simulink model "propeller"  (R2019b)
settings: Solver=VariableStepAuto  StartTime=0.0  StopTime=180  MaxStep=1e-2  RelTol=1e-3
undefined symbols (not defined in the file or in its folder): X, Y, Z
libraries: sm_lib x26, cstblocks x23, nesl_utility x20, simulink x2
(part 1 of 3)
settings Model: PauseTimes=1.42  EnablePacing=on  Creator=lenovo  LastModifiedBy=lenovo

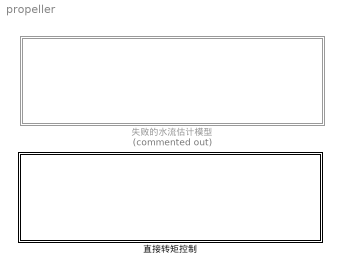
== system propeller ==
  失败的水流估计模型 : Subsystem  Commented=on
  直接转矩控制 : Subsystem

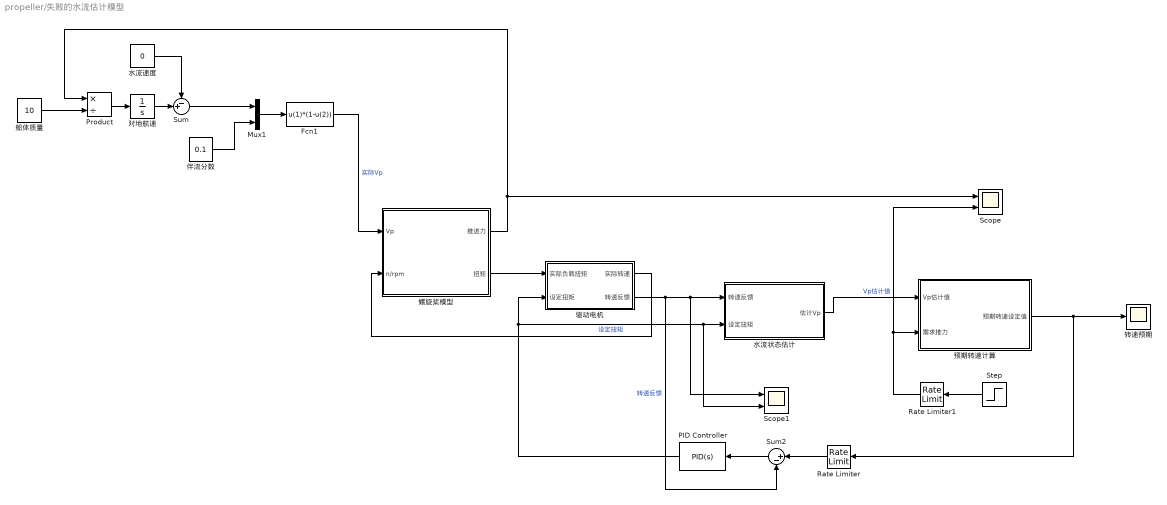
== system propeller/失败的水流估计模型 ==
  Fcn1 : Fcn  Expr=u(1)*(1-u(2))
  Mux1 : Mux  Inputs=2
  PID Controller : simulink/Continuous/PID Controller  Controller=PID  Form=Parallel  TimeDomain=Continuous-time  SampleTime=-1  IntegratorMethod=Forward Euler  FilterMethod=Forward Euler  ControllerParametersSource=internal  P=0.05  I=0.01  D=0  UseFilter=on  N=100  TunerSelectOption=Transfer Function Based (PID Tuner App)  InitialConditionSource=internal  InitialConditionForIntegrator=0  InitialConditionForFilter=0  DifferentiatorICPrevScaledInput=0  ExternalReset=none  TrackingMode=off  Kt=1  LimitOutput=on  UpperSaturationLimit=250  LowerSaturationLimit=-250  LinearizeAsGain=on  AntiWindupMode=none  Kb=1  POutMin=[]  POutMax=[]  IOutMin=[]  IOutMax=[]  DOutMin=[]  DOutMax=[]  NOutMin=[]  NOutMax=[]  SumOutMin=[]  SumOutMax=[]  SaturationOutMin=[]  SaturationOutMax=[]  PParamMin=[]  PParamMax=[]  IParamMin=[]  IParamMax=[]  DParamMin=[]  DParamMax=[]  NParamMin=[]  NParamMax=[]  KbParamMin=[]  KbParamMax=[]  KtParamMin=[]  KtParamMax=[]  KbOutMin=[]  KbOutMax=[]  KtOutMin=[]  KtOutMax=[]  IntegratorOutMin=[]  IntegratorOutMax=[]  FilterOutMin=[]  FilterOutMax=[]  SumI1OutMin=[]  SumI1OutMax=[]  SumI2OutMin=[]  SumI2OutMax=[]  SumI3OutMin=[]  SumI3OutMax=[]  SumI4OutMin=[]  SumI4OutMax=[]  SumDOutMin=[]  SumDOutMax=[]  DifferentiatorOutMin=[]  DifferentiatorOutMax=[]  FilterDiffOutCoefMin=[]  FilterDiffOutCoefMax=[]  ReciprocalOutMin=[]  ReciprocalOutMax=[]  SumDenOutMin=[]  SumDenOutMax=[]  SumNumOutMin=[]  SumNumOutMax=[]  DivideOutMin=[]  DivideOutMax=[]  IntegratorContinuousStateAttributes=''  IntegratorStateMustResolveToSignalObject=off  IntegratorRTWStateStorageClass=Auto  FilterContinuousStateAttributes=''  FilterStateMustResolveToSignalObject=off  FilterRTWStateStorageClass=Auto  ParallelPVariant=InternalParameters  IdealPVariant=Disabled  IVariant=InternalParameters  DVariant=InternalParameters  IntegratorVariant=Continuous  SatVariant=Enabled  AWVariant=Passthrough  PCopyVariant=Disabled  TRVariant=Disabled  FdbkBlocksVariant=Forward  IdealPFdbkVariant=Disabled  SatFdbkVariant=Disabled  DerivativeFilterVariant=ContFilter  NVariant=InternalParameters  NCopyVariant=Disabled  FilterICVariant=InternalICsFilter  IntegratorICVariant=InternalICs  ExternalResetVariant=Disabled  TRSumVariant=Passthrough  SumFdbkVariant=Disabled  SumVariant=Sum_PID
  Product : Product  Inputs=*/
  Rate Limiter : RateLimiter  RisingSlewLimit=200  FallingSlewLimit=-200  SampleTimeMode=inherited
  Rate Limiter1 : RateLimiter  RisingSlewLimit=3  FallingSlewLimit=-3  SampleTimeMode=inherited
  Scope : Scope  NumInputPorts=2
  Scope1 : Scope  NumInputPorts=2
  Step : Step  Time=5  Before=1  After=3  SampleTime=0
  Sum : Sum  Inputs=-+|
  Sum2 : Sum  Inputs=|+-
  伴流分数 : Constant  Value=0.1
  对地航速 : Integrator
  水流状态估计 : Subsystem
  水流速度 : Constant  Value=0
  船体质量 : Constant  Value=10
  螺旋桨模型 : Subsystem  mask{rou_Set=1.023, D_Set=1}
      mask prompts: rou_Set "海水密度 g/cm3 (rou_Set)"; D_Set "螺旋桨直径 D_Set"
  转速预期 : Scope
  预期转速计算 : Subsystem
  驱动电机 : Subsystem  mask{Trq_Max=250, Spe_Max=20000, J_Set=0.1}
      mask prompts: Trq_Max "电机最大扭矩"; Spe_Max "电机最高转速"; J_Set "系统转动惯量"
  wires:
  驱动电机/2(转速反馈) -> Sum2/2, Scope1/1, 水流状态估计/1(转速反馈)  "转速反馈"
  PID Controller/1 -> 驱动电机/2(设定扭矩), Scope1/2, 水流状态估计/2(设定扭矩)  "设定扭矩"
  螺旋桨模型/2(扭矩) -> 驱动电机/1(实际负载扭矩)
  Product/1 -> 对地航速/1
  Rate Limiter1/1 -> Scope/2, 预期转速计算/2(需求推力)
  水流状态估计/1(估计Vp) -> 预期转速计算/1(Vp估计值)  "Vp估计值"
  驱动电机/1(实际转速) -> 螺旋桨模型/2(n/rpm)
  Sum/1 -> Mux1/1
  Sum2/1 -> PID Controller/1
  Fcn1/1 -> 螺旋桨模型/1(Vp)  "实际Vp"
  Step/1 -> Rate Limiter1/1
  对地航速/1 -> Sum/2
  Rate Limiter/1 -> Sum2/1
  预期转速计算/1(预期转速设定值) -> Rate Limiter/1, 转速预期/1
  螺旋桨模型/1(推进力) -> Product/1, Scope/1
  Mux1/1 -> Fcn1/1
  伴流分数/1 -> Mux1/2
  船体质量/1 -> Product/2
  水流速度/1 -> Sum/1

== system propeller/直接转矩控制 ==
  Constant2 : Constant  Value=60
  Constant3 : Constant  Value=2.5
  GPS船速 : Subsystem
  Rate Limiter1 : RateLimiter  RisingSlewLimit=2  FallingSlewLimit=-2  SampleTimeMode=inherited
  Slider : SliderBlock  ScaleMin=-60  ScaleMax=60
  保证初始设定值为0 : TransportDelay  DelayTime=0.01
  船体、水体物理模型 : Subsystem
  船速、朝向控制器 : Subsystem
  wires:
  GPS船速/1(纵向速度) -> 船速、朝向控制器/5(前进速度反馈)
  GPS船速/2(横向速度) -> 船速、朝向控制器/6(侧移速度反馈)
  船体、水体物理模型/3(Angle) -> 船速、朝向控制器/7(角度反馈), GPS船速/3(Alpha)
  船速、朝向控制器/1(左推进方向) -> 船体、水体物理模型/1(左推进方向设定)
  船速、朝向控制器/2(右推进方向) -> 船体、水体物理模型/2(右推进方向设定)
  船速、朝向控制器/3(左电机扭矩) -> 船体、水体物理模型/3(左设定扭矩)
  船速、朝向控制器/4(右电机扭矩) -> 船体、水体物理模型/4(右设定扭矩)
  船体、水体物理模型/4(左转速反馈) -> 船速、朝向控制器/1(左电机转速反馈)
  船体、水体物理模型/5(实际推进方向) -> 船速、朝向控制器/2(推进方向反馈)
  船体、水体物理模型/6(右转速反馈) -> 船速、朝向控制器/3(右电机转速反馈)
  船体、水体物理模型/7(wz) -> 船速、朝向控制器/4(角速度反馈)
  船体、水体物理模型/8(Vx) -> GPS船速/1(Vx)
  船体、水体物理模型/9(Vy) -> GPS船速/2(Vy)
  Rate Limiter1/1 -> 船速、朝向控制器/8(船头方向设定)
  Constant2/1 -> 保证初始设定值为0/1
  保证初始设定值为0/1 -> Rate Limiter1/1
  Constant3/1 -> 船速、朝向控制器/9(前进速度设定)

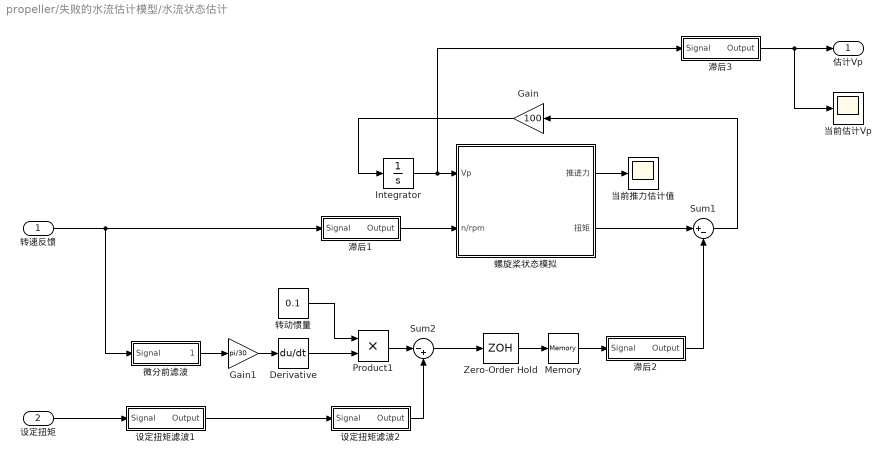
== system propeller/失败的水流估计模型/水流状态估计 ==
  转速反馈 : Inport
  设定扭矩 : Inport  Port=2
  Derivative : Derivative  CoefficientInTFapproximation=1/25
  Gain : Gain  Gain=100
  Gain1 : Gain  Gain=pi/30
  Integrator : Integrator  LimitOutput=on  UpperSaturationLimit=20  LowerSaturationLimit=-20
  Memory : Memory
  Product1 : Product
  Sum1 : Sum  Inputs=|+-
  Sum2 : Sum  Inputs=|-+
  Zero-Order Hold : ZeroOrderHold  SampleTime=0.01
  当前估计Vp : Scope
  当前推力估计值 : Scope
  微分前滤波 : Subsystem  mask{Frq=10, Order=1}
      mask prompts: Frq "Frq_Set"; Order "Order_Set"
  滞后1 : Subsystem  mask{Frq=5, Order=1}
      mask prompts: Frq "Frq_Set"; Order "Order_Set"
  滞后2 : Subsystem  mask{Frq=5, Order=1}
      mask prompts: Frq "Frq_Set"; Order "Order_Set"
  滞后3 : Subsystem  mask{Frq=2, Order=10}
      mask prompts: Frq "Frq_Set"; Order "Order_Set"
  螺旋桨状态模拟 : Subsystem  mask{rou_Set=1.023, D_Set=1}
      mask prompts: rou_Set "海水密度 g/cm3 (rou_Set)"; D_Set "螺旋桨直径 D_Set"
  设定扭矩滤波1 : Subsystem  mask{Frq=25, Order=1}
      mask prompts: Frq "Frq_Set"; Order "Order_Set"
  设定扭矩滤波2 : Subsystem  mask{Frq=10, Order=1}
      mask prompts: Frq "Frq_Set"; Order "Order_Set"
  转动惯量 : Constant  Value=0.1
  估计Vp : Outport
  wires:
  微分前滤波/1(Output) -> Gain1/1
  Gain1/1 -> Derivative/1
  Product1/1 -> Sum2/1
  螺旋桨状态模拟/2(扭矩) -> Sum1/1
  转速反馈/1 -> 微分前滤波/1(Signal), 滞后1/1(Signal)
  滞后2/1(Output) -> Sum1/2
  转动惯量/1 -> Product1/1
  Derivative/1 -> Product1/2
  滞后1/1(Output) -> 螺旋桨状态模拟/2(n/rpm)
  螺旋桨状态模拟/1(推进力) -> 当前推力估计值/1
  设定扭矩滤波1/1(Output) -> 设定扭矩滤波2/1(Signal)
  Gain/1 -> Integrator/1
  设定扭矩滤波2/1(Output) -> Sum2/2
  滞后3/1(Output) -> 当前估计Vp/1, 估计Vp/1
  Sum2/1 -> Zero-Order Hold/1
  设定扭矩/1 -> 设定扭矩滤波1/1(Signal)
  Sum1/1 -> Gain/1
  Integrator/1 -> 滞后3/1(Signal), 螺旋桨状态模拟/1(Vp)
  Zero-Order Hold/1 -> Memory/1
  Memory/1 -> 滞后2/1(Signal)

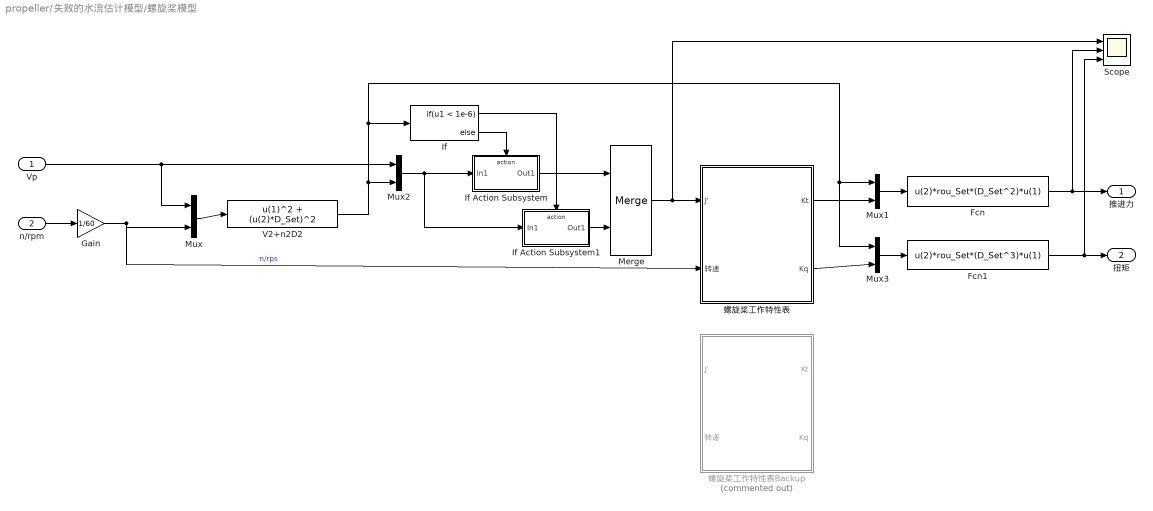
== system propeller/失败的水流估计模型/螺旋桨模型 ==
  Vp : Inport
  n/rpm : Inport  Port=2
  Fcn : Fcn  Expr=u(2)*rou_Set*(D_Set^2)*u(1)
  Fcn1 : Fcn  Expr=u(2)*rou_Set*(D_Set^3)*u(1)
  Gain : Gain  Gain=1/60
  If : If  IfExpression=u1 < 1e-6
  If Action Subsystem : Subsystem  TreatAsAtomicUnit=on
  If Action Subsystem1 : Subsystem  TreatAsAtomicUnit=on
  Merge : Merge
  Mux{,1..3} (4 alike) : Mux  Inputs=2
  Scope : Scope  NumInputPorts=3
  V2+n2D2 : Fcn  Expr=u(1)^2 + (u(2)*D_Set)^2
  螺旋桨工作特性表 : Subsystem
  螺旋桨工作特性表Backup : Subsystem  Commented=on
  推进力 : Outport
  扭矩 : Outport  Port=2
  wires:
  Mux2/1 -> If Action Subsystem1/1(In1), If Action Subsystem/1(In1)
  n/rpm/1 -> Gain/1
  Vp/1 -> Mux2/1, Mux/1
  If/2 -> If Action Subsystem/Action
  If Action Subsystem/1(Out1) -> Merge/1
  Gain/1 -> 螺旋桨工作特性表/2(转速), Mux/2  "n/rps"
  If/1 -> If Action Subsystem1/Action
  If Action Subsystem1/1(Out1) -> Merge/2
  Mux/1 -> V2+n2D2/1
  Merge/1 -> Scope/1, 螺旋桨工作特性表/1(J')
  螺旋桨工作特性表/1(Kt) -> Mux1/2
  螺旋桨工作特性表/2(Kq) -> Mux3/2
  Mux1/1 -> Fcn/1
  V2+n2D2/1 -> If/1, Mux3/1, Mux1/1, Mux2/2
  Mux3/1 -> Fcn1/1
  Fcn1/1 -> Scope/3, 扭矩/1
  Fcn/1 -> Scope/2, 推进力/1

== system propeller/失败的水流估计模型/预期转速计算 ==
  Vp估计值 : Inport
  需求推力 : Inport  Port=2
  Gain : Gain  Gain=1000
  Integrator : Integrator
  Sum1 : Sum  Inputs=+-|
  当前扭矩估计值 : Scope
  滞后2 : Subsystem  mask{Frq=0.2, Order=5}
      mask prompts: Frq "Frq_Set"; Order "Order_Set"
  螺旋桨状态模拟 : Subsystem  mask{rou_Set=1.023, D_Set=1}
      mask prompts: rou_Set "海水密度 g/cm3 (rou_Set)"; D_Set "螺旋桨直径 D_Set"
  预期转速设定值 : Outport
  wires:
  螺旋桨状态模拟/1(推进力) -> Sum1/2
  Gain/1 -> Integrator/1
  Integrator/1 -> 滞后2/1(Signal), 螺旋桨状态模拟/2(n/rpm)
  Sum1/1 -> Gain/1
  螺旋桨状态模拟/2(扭矩) -> 当前扭矩估计值/1
  需求推力/1 -> Sum1/1
  Vp估计值/1 -> 螺旋桨状态模拟/1(Vp)
  滞后2/1(Output) -> 预期转速设定值/1

== system propeller/失败的水流估计模型/驱动电机 ==
  实际负载扭矩 : Inport
  设定扭矩 : Inport  Port=2
  Gain : Gain  Gain=30/pi
  Integrator : Integrator  LimitOutput=on  UpperSaturationLimit=5000  LowerSaturationLimit=-5000
  Product1 : Product  Inputs=/*
  Saturation : Saturate  UpperLimit=Trq_Max  LowerLimit=-Trq_Max
  Sum1 : Sum  Inputs=|+-
  传感器量化 : Quantizer  QuantizationInterval=Spe_Max/10000
  反馈量滤波 : Subsystem  mask{Frq=25, Order=3}
      mask prompts: Frq "Frq_Set"; Order "Order_Set"
  滞后 : Subsystem  mask{Frq=500, Order=2}
      mask prompts: Frq "Frq_Set"; Order "Order_Set"
  转动惯量 : Constant  Value=J_Set
  通信量化 : Quantizer  QuantizationInterval=Trq_Max/5000
  通信间隔 : ZeroOrderHold  SampleTime=0.01
  实际转速 : Outport
  转速反馈 : Outport  Port=2
  wires:
  通信量化/1 -> Saturation/1
  Sum1/1 -> Product1/2
  通信间隔/1 -> 反馈量滤波/1(Signal)
  传感器量化/1 -> 通信间隔/1
  转动惯量/1 -> Product1/1
  实际负载扭矩/1 -> Sum1/2
  Saturation/1 -> 滞后/1(Signal)
  Product1/1 -> Integrator/1
  滞后/1(Output) -> Sum1/1
  Integrator/1 -> Gain/1  "n_Radps"
  设定扭矩/1 -> 通信量化/1
  反馈量滤波/1(Output) -> 转速反馈/1
  Gain/1 -> 实际转速/1, 传感器量化/1

== system propeller/直接转矩控制/GPS船速 ==
  Vx : Inport
  Vy : Inport  Port=2
  Alpha : Inport  Port=3
  Fcn1 : Fcn  Expr=u(2)*cos(u(3))-u(1)*sin(u(3))
  Fcn2 : Fcn  Expr=u(2)*sin(u(3))+u(1)*cos(u(3))
  Mux1 : Mux  Inputs=3
  传感器量化 : Quantizer  QuantizationInterval=0.01
  传感器量化1 : Quantizer  QuantizationInterval=0.01
  反馈量滤波 : Subsystem  mask{Frq=1, Order=3}
      mask prompts: Frq "Frq_Set"; Order "Order_Set"
  反馈量滤波1 : Subsystem  mask{Frq=1, Order=3}
      mask prompts: Frq "Frq_Set"; Order "Order_Set"
  通信间隔 : ZeroOrderHold  SampleTime=0.01
  通信间隔1 : ZeroOrderHold  SampleTime=0.01
  纵向速度 : Outport
  横向速度 : Outport  Port=2
  wires:
  Fcn1/1 -> 传感器量化/1
  Alpha/1 -> Mux1/3
  Vx/1 -> Mux1/1
  Vy/1 -> Mux1/2
  Mux1/1 -> Fcn1/1, Fcn2/1
  传感器量化/1 -> 通信间隔/1
  反馈量滤波/1(Output) -> 纵向速度/1
  通信间隔/1 -> 反馈量滤波/1(Signal)
  通信间隔1/1 -> 反馈量滤波1/1(Signal)
  传感器量化1/1 -> 通信间隔1/1
  Fcn2/1 -> 传感器量化1/1
  反馈量滤波1/1(Output) -> 横向速度/1

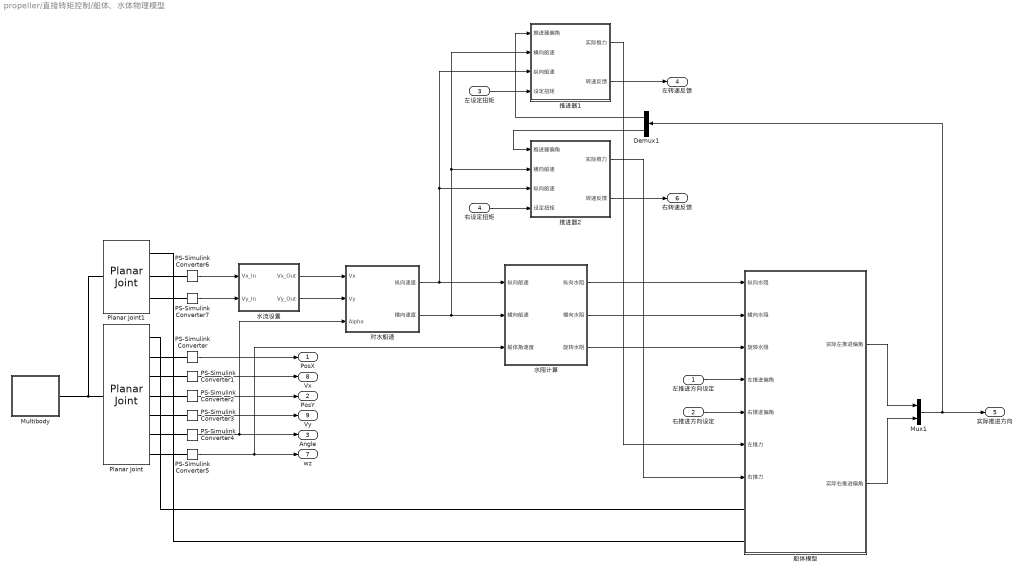
== system propeller/直接转矩控制/船体、水体物理模型 ==
  左推进方向设定 : Inport
  右推进方向设定 : Inport  Port=2
  左设定扭矩 : Inport  Port=3
  右设定扭矩 : Inport  Port=4
  Demux1 : Demux  Outputs=2
  Multibody : Subsystem
  Mux1 : Mux  Inputs=2
  PS-Simulink Converter{,1..7} (8 alike) : nesl_utility/PS-Simulink Converter  PhysicalDomain=network_engine_domain  SubClassName=ps_output  LeftPortType=input  RightPortType=output  PseudoPeriodic=off  Frequencies=[]  Unit=inherit  AffineConversion=off
  Planar Joint : sm_lib/Joints/Planar Joint  JointMode=Normal  SenseConstraintForce=off  SenseConstraintForceX=off  SenseConstraintForceY=off  SenseConstraintForceZ=off  SenseConstraintTorque=off  SenseConstraintTorqueX=off  SenseConstraintTorqueY=off  SenseConstraintTorqueZ=off  SenseTotalForce=off  SenseTotalForceX=off  SenseTotalForceY=off  SenseTotalForceZ=off  SenseTotalTorque=off  SenseTotalTorqueX=off  SenseTotalTorqueY=off  SenseTotalTorqueZ=off  CompositeWrenchDir=FollowerOnBase  CompositeWrenchFrame=BaseFrame  PxEquilibriumPosition=0  PxEquilibriumPositionUnits=m  PxSpringStiffness=0  PxSpringStiffnessUnits=N/m  PxDampingCoefficient=0  PxDampingCoefficientUnits=N/(m/s)  PxTorqueActuationMode=NoTorque  PxMotionActuationMode=ComputedMotion  PxSensePosition=on  PxSenseVelocity=on  PxSenseAcceleration=off  PxSenseTorqueForce=off  PxSenseLowerLimitTorqueForce=off  PxSenseUpperLimitTorqueForce=off  PxLowerLimitSpecify=off  PxLowerLimitBound=-1  PxLowerLimitBoundUnits=m  PxLowerLimitStiffness=1e6  PxLowerLimitStiffnessUnits=N/m  PxLowerLimitDamping=1e3  PxLowerLimitDampingUnits=N/(m/s)  PxLowerLimitTransitionRegionWidth=1e-4  PxLowerLimitTransitionRegionWidthUnits=m  PxUpperLimitSpecify=off  PxUpperLimitBound=1  PxUpperLimitBoundUnits=m  PxUpperLimitStiffness=1e6  PxUpperLimitStiffnessUnits=N/m  PxUpperLimitDamping=1e3  PxUpperLimitDampingUnits=N/(m/s)  PxUpperLimitTransitionRegionWidth=1e-4  PxUpperLimitTransitionRegionWidthUnits=m  PxPositionTargetSpecify=off  PxPositionTargetPriority=High  PxPositionTargetValue=0  PxPositionTargetValueUnits=m  PxVelocityTargetSpecify=off  PxVelocityTargetPriority=High  PxVelocityTargetValue=3  PxVelocityTargetValueUnits=m/s  PyEquilibriumPosition=0  PyEquilibriumPositionUnits=m  PySpringStiffness=0  PySpringStiffnessUnits=N/m  PyDampingCoefficient=0  PyDampingCoefficientUnits=N/(m/s)  PyTorqueActuationMode=NoTorque  PyMotionActuationMode=ComputedMotion  PySensePosition=on  PySenseVelocity=on  PySenseAcceleration=off  PySenseTorqueForce=off  PySenseLowerLimitTorqueForce=off  PySenseUpperLimitTorqueForce=off  PyLowerLimitSpecify=off  PyLowerLimitBound=-1  PyLowerLimitBoundUnits=m  PyLowerLimitStiffness=1e6  PyLowerLimitStiffnessUnits=N/m  PyLowerLimitDamping=1e3  PyLowerLimitDampingUnits=N/(m/s)  PyLowerLimitTransitionRegionWidth=1e-4  PyLowerLimitTransitionRegionWidthUnits=m  PyUpperLimitSpecify=off  PyUpperLimitBound=1  PyUpperLimitBoundUnits=m  PyUpperLimitStiffness=1e6  PyUpperLimitStiffnessUnits=N/m  PyUpperLimitDamping=1e3  PyUpperLimitDampingUnits=N/(m/s)  PyUpperLimitTransitionRegionWidth=1e-4  PyUpperLimitTransitionRegionWidthUnits=m  PyPositionTargetSpecify=off  PyPositionTargetPriority=High  PyPositionTargetValue=0  PyPositionTargetValueUnits=m  PyVelocityTargetSpecify=off  PyVelocityTargetPriority=High  PyVelocityTargetValue=1  PyVelocityTargetValueUnits=m/s  RzEquilibriumPosition=0  RzEquilibriumPositionUnits=deg  RzSpringStiffness=0  RzSpringStiffnessUnits=N*m/deg  RzDampingCoefficient=0  RzDampingCoefficientUnits=N*m/(deg/s)  RzTorqueActuationMode=NoTorque  RzMotionActuationMode=ComputedMotion  RzSensePosition=on  RzSenseVelocity=on  RzSenseAcceleration=off  RzSenseTorqueForce=off  RzSenseLowerLimitTorqueForce=off  RzSenseUpperLimitTorqueForce=off  RzLowerLimitSpecify=off  RzLowerLimitBound=-90  RzLowerLimitBoundUnits=deg  RzLowerLimitStiffness=1e4  RzLowerLimitStiffnessUnits=N*m/deg  RzLowerLimitDamping=10  RzLowerLimitDampingUnits=N*m/(deg/s)  RzLowerLimitTransitionRegionWidth=0.1  RzLowerLimitTransitionRegionWidthUnits=deg  RzUpperLimitSpecify=off  RzUpperLimitBound=90  RzUpperLimitBoundUnits=deg  RzUpperLimitStiffness=1e4  RzUpperLimitStiffnessUnits=N*m/deg  RzUpperLimitDamping=10  RzUpperLimitDampingUnits=N*m/(deg/s)  RzUpperLimitTransitionRegionWidth=0.1  RzUpperLimitTransitionRegionWidthUnits=deg  RzPositionTargetSpecify=off  RzPositionTargetPriority=High  RzPositionTargetValue=0  RzPositionTargetValueUnits=deg  RzVelocityTargetSpecify=off  RzVelocityTargetPriority=High  RzVelocityTargetValue=0  RzVelocityTargetValueUnits=deg/s
  Planar Joint1 : sm_lib/Joints/Planar Joint  JointMode=Normal  SenseConstraintForce=off  SenseConstraintForceX=off  SenseConstraintForceY=off  SenseConstraintForceZ=off  SenseConstraintTorque=off  SenseConstraintTorqueX=off  SenseConstraintTorqueY=off  SenseConstraintTorqueZ=off  SenseTotalForce=off  SenseTotalForceX=off  SenseTotalForceY=off  SenseTotalForceZ=off  SenseTotalTorque=off  SenseTotalTorqueX=off  SenseTotalTorqueY=off  SenseTotalTorqueZ=off  CompositeWrenchDir=FollowerOnBase  CompositeWrenchFrame=BaseFrame  PxEquilibriumPosition=0  PxEquilibriumPositionUnits=m  PxSpringStiffness=0  PxSpringStiffnessUnits=N/m  PxDampingCoefficient=0  PxDampingCoefficientUnits=N/(m/s)  PxTorqueActuationMode=NoTorque  PxMotionActuationMode=ComputedMotion  PxSensePosition=off  PxSenseVelocity=on  PxSenseAcceleration=off  PxSenseTorqueForce=off  PxSenseLowerLimitTorqueForce=off  PxSenseUpperLimitTorqueForce=off  PxLowerLimitSpecify=off  PxLowerLimitBound=-1  PxLowerLimitBoundUnits=m  PxLowerLimitStiffness=1e6  PxLowerLimitStiffnessUnits=N/m  PxLowerLimitDamping=1e3  PxLowerLimitDampingUnits=N/(m/s)  PxLowerLimitTransitionRegionWidth=1e-4  PxLowerLimitTransitionRegionWidthUnits=m  PxUpperLimitSpecify=off  PxUpperLimitBound=1  PxUpperLimitBoundUnits=m  PxUpperLimitStiffness=1e6  PxUpperLimitStiffnessUnits=N/m  PxUpperLimitDamping=1e3  PxUpperLimitDampingUnits=N/(m/s)  PxUpperLimitTransitionRegionWidth=1e-4  PxUpperLimitTransitionRegionWidthUnits=m  PxPositionTargetSpecify=off  PxPositionTargetPriority=High  PxPositionTargetValue=0  PxPositionTargetValueUnits=m  PxVelocityTargetSpecify=off  PxVelocityTargetPriority=High  PxVelocityTargetValue=3  PxVelocityTargetValueUnits=m/s  PyEquilibriumPosition=0  PyEquilibriumPositionUnits=m  PySpringStiffness=0  PySpringStiffnessUnits=N/m  PyDampingCoefficient=0  PyDampingCoefficientUnits=N/(m/s)  PyTorqueActuationMode=NoTorque  PyMotionActuationMode=ComputedMotion  PySensePosition=off  PySenseVelocity=on  PySenseAcceleration=off  PySenseTorqueForce=off  PySenseLowerLimitTorqueForce=off  PySenseUpperLimitTorqueForce=off  PyLowerLimitSpecify=off  PyLowerLimitBound=-1  PyLowerLimitBoundUnits=m  PyLowerLimitStiffness=1e6  PyLowerLimitStiffnessUnits=N/m  PyLowerLimitDamping=1e3  PyLowerLimitDampingUnits=N/(m/s)  PyLowerLimitTransitionRegionWidth=1e-4  PyLowerLimitTransitionRegionWidthUnits=m  PyUpperLimitSpecify=off  PyUpperLimitBound=1  PyUpperLimitBoundUnits=m  PyUpperLimitStiffness=1e6  PyUpperLimitStiffnessUnits=N/m  PyUpperLimitDamping=1e3  PyUpperLimitDampingUnits=N/(m/s)  PyUpperLimitTransitionRegionWidth=1e-4  PyUpperLimitTransitionRegionWidthUnits=m  PyPositionTargetSpecify=off  PyPositionTargetPriority=High  PyPositionTargetValue=0  PyPositionTargetValueUnits=m  PyVelocityTargetSpecify=off  PyVelocityTargetPriority=High  PyVelocityTargetValue=1  PyVelocityTargetValueUnits=m/s  RzEquilibriumPosition=0  RzEquilibriumPositionUnits=deg  RzSpringStiffness=0  RzSpringStiffnessUnits=N*m/deg  RzDampingCoefficient=0  RzDampingCoefficientUnits=N*m/(deg/s)  RzTorqueActuationMode=NoTorque  RzMotionActuationMode=ComputedMotion  RzSensePosition=off  RzSenseVelocity=off  RzSenseAcceleration=off  RzSenseTorqueForce=off  RzSenseLowerLimitTorqueForce=off  RzSenseUpperLimitTorqueForce=off  RzLowerLimitSpecify=off  RzLowerLimitBound=-90  RzLowerLimitBoundUnits=deg  RzLowerLimitStiffness=1e4  RzLowerLimitStiffnessUnits=N*m/deg  RzLowerLimitDamping=10  RzLowerLimitDampingUnits=N*m/(deg/s)  RzLowerLimitTransitionRegionWidth=0.1  RzLowerLimitTransitionRegionWidthUnits=deg  RzUpperLimitSpecify=off  RzUpperLimitBound=90  RzUpperLimitBoundUnits=deg  RzUpperLimitStiffness=1e4  RzUpperLimitStiffnessUnits=N*m/deg  RzUpperLimitDamping=10  RzUpperLimitDampingUnits=N*m/(deg/s)  RzUpperLimitTransitionRegionWidth=0.1  RzUpperLimitTransitionRegionWidthUnits=deg  RzPositionTargetSpecify=off  RzPositionTargetPriority=High  RzPositionTargetValue=0  RzPositionTargetValueUnits=deg  RzVelocityTargetSpecify=off  RzVelocityTargetPriority=High  RzVelocityTargetValue=0  RzVelocityTargetValueUnits=deg/s
  对水船速 : Subsystem
  推进器1 : Subsystem
  推进器2 : Subsystem
  水流设置 : Subsystem  mask{Spe=0, Dir=90}
      mask prompts: Spe "水流流速  m/s"; Dir "水流角度 度 0度对应+X"
  水阻计算 : Subsystem  mask{K_y=8, K_x=100, K_z=15000}
      mask prompts: K_y "前进水阻力系数"; K_x "侧移水阻力系数"; K_z "自旋水阻力系数"
  船体模型 : Subsystem  mask{M_Set=1500}
      mask prompts: M_Set "船体质量"
  PosX : Outport
  PosY : Outport  Port=2
  Angle : Outport  Port=3
  左转速反馈 : Outport  Port=4
  实际推进方向 : Outport  Port=5
  右转速反馈 : Outport  Port=6
  wz : Outport  Port=7
  Vx : Outport  Port=8
  Vy : Outport  Port=9
  wires:
  PS-Simulink Converter1/1 -> Vx/1
  推进器1/1(实际推力) -> 船体模型/6(左推力)
  水流设置/1(Vx_Out) -> 对水船速/1(Vx)
  对水船速/2(横向速度) -> 推进器1/2(横向船速), 推进器2/2(横向船速), 水阻计算/2(横向船速)
  推进器1/2(转速反馈) -> 左转速反馈/1
  PS-Simulink Converter5/1 -> wz/1, 水阻计算/3(船体角速度)
  对水船速/1(纵向速度) -> 推进器1/3(纵向船速), 推进器2/3(纵向船速), 水阻计算/1(纵向船速)
  水阻计算/2(横向水阻) -> 船体模型/2(横向水阻)
  推进器2/2(转速反馈) -> 右转速反馈/1
  PS-Simulink Converter/1 -> PosX/1
  左推进方向设定/1 -> 船体模型/4(左推进偏角)
  左设定扭矩/1 -> 推进器1/4(设定扭矩)
  PS-Simulink Converter3/1 -> Vy/1
  PS-Simulink Converter6/1 -> 水流设置/1(Vx_In)
  水流设置/2(Vy_Out) -> 对水船速/2(Vy)
  水阻计算/1(纵向水阻) -> 船体模型/1(纵向水阻)
  Mux1/1 -> Demux1/1, 实际推进方向/1
  水阻计算/3(旋转水阻) -> 船体模型/3(旋转水阻)
  PS-Simulink Converter2/1 -> PosY/1
  PS-Simulink Converter4/1 -> Angle/1, 对水船速/3(Alpha)
  推进器2/1(实际推力) -> 船体模型/7(右推力)
  PS-Simulink Converter7/1 -> 水流设置/2(Vy_In)
  右推进方向设定/1 -> 船体模型/5(右推进偏角)
  右设定扭矩/1 -> 推进器2/4(设定扭矩)
  船体模型/1(实际左推进偏角) -> Mux1/1
  船体模型/2(实际右推进偏角) -> Mux1/2
  Demux1/1 -> 推进器1/1(推进器偏角)
  Demux1/2 -> 推进器2/1(推进器偏角)
  connections:
  PS-Simulink Converter/LConn1 -- Planar Joint/RConn2
  PS-Simulink Converter7/LConn1 -- Planar Joint1/RConn3
  PS-Simulink Converter5/LConn1 -- Planar Joint/RConn7
  PS-Simulink Converter2/LConn1 -- Planar Joint/RConn4
  PS-Simulink Converter4/LConn1 -- Planar Joint/RConn6
  Planar Joint/LConn1 -- Planar Joint1/LConn1 -- Multibody/RConn1
  船体模型/LConn1 -- Planar Joint/RConn1
  PS-Simulink Converter6/LConn1 -- Planar Joint1/RConn2
  PS-Simulink Converter1/LConn1 -- Planar Joint/RConn3
  PS-Simulink Converter3/LConn1 -- Planar Joint/RConn5
  Planar Joint1/RConn1 -- 船体模型/LConn2

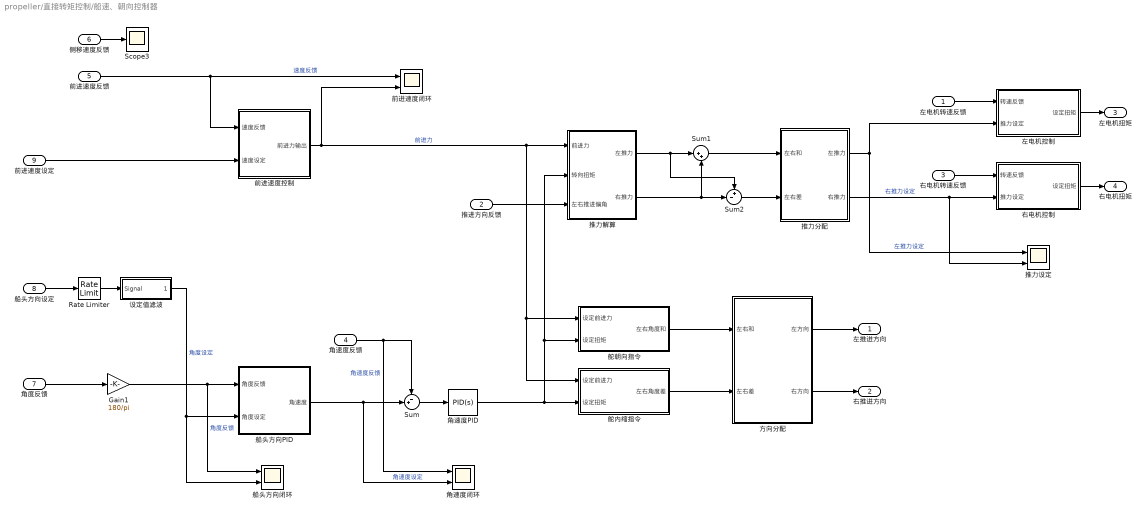
== system propeller/直接转矩控制/船速、朝向控制器 ==
  左电机转速反馈 : Inport
  推进方向反馈 : Inport  Port=2
  右电机转速反馈 : Inport  Port=3
  角速度反馈 : Inport  Port=4
  前进速度反馈 : Inport  Port=5
  侧移速度反馈 : Inport  Port=6
  角度反馈 : Inport  Port=7
  船头方向设定 : Inport  Port=8
  前进速度设定 : Inport  Port=9
  Gain1 : Gain  Gain=180/pi
  Rate Limiter : RateLimiter  RisingSlewLimit=5  FallingSlewLimit=-5  SampleTimeMode=inherited
  Scope3 : Scope
  Sum : Sum  Inputs=-+|
  Sum1 : Sum  Inputs=|++
  Sum2 : Sum  Inputs=+-|
  前进速度控制 : Subsystem  mask{Trq_p=50, Trq_n=50, Kp=250, Ki=4, Kd=8, D_Fc=1}
      mask prompts: Trq_p "最大推进扭矩"; Trq_n "最大制动扭矩"; Kp "PID-P"; Ki "PID-I"; Kd "PID-D"; D_Fc "PID-微分截止频率"
  前进速度闭环 : Scope  NumInputPorts=2
  右电机控制 : Subsystem
  左电机控制 : Subsystem
  推力分配 : Subsystem  mask{Max_Trq=25}
      mask prompts: Max_Trq "单侧最高扭矩"
  推力解算 : Subsystem  mask{a=1, b=3}
      mask prompts: a "推进器安装横向距离 a"; b "推进器安装纵向距离 b"
  推力设定 : Scope  NumInputPorts=2
  方向分配 : Subsystem  mask{Max_Th=30}
      mask prompts: Max_Th "单侧最大角度"
  舵内缩指令 : Subsystem  mask{Th_Max=30, Fy_Start=10, Trq_Start=25}
      mask prompts: Th_Max "单侧最大偏角"; Fy_Start "启用舵内缩的最大前进推力"; Trq_Start "启用舵内缩的扭矩差"
  舵朝向指令 : Subsystem  mask{Th_Max=30, Fy_Start=10}
      mask prompts: Th_Max "单侧最大偏角"; Fy_Start "启用舵转向的最小前进推力"
  船头方向PID : Subsystem  mask{Spe_p=30, Spe_n=30, Kp=2, Ki=0, Kd=3, D_Fc=5}
      mask prompts: Spe_p "最大左转角速度 dps"; Spe_n "最大右转角速度 dps"; Kp "PID-P"; Ki "PID-I"; Kd "PID-D"; D_Fc "PID-微分截止频率"
  船头方向闭环 : Scope  NumInputPorts=2
  角速度PID : simulink/Continuous/PID Controller  Controller=PID  Form=Parallel  TimeDomain=Continuous-time  SampleTime=-1  IntegratorMethod=Forward Euler  FilterMethod=Forward Euler  ControllerParametersSource=internal  P=350  I=0  D=150  UseFilter=on  N=10  TunerSelectOption=Transfer Function Based (PID Tuner App)  InitialConditionSource=internal  InitialConditionForIntegrator=0  InitialConditionForFilter=0  DifferentiatorICPrevScaledInput=0  ExternalReset=none  TrackingMode=off  Kt=1  LimitOutput=off  UpperSaturationLimit=inf  LowerSaturationLimit=-inf  LinearizeAsGain=on  AntiWindupMode=none  Kb=1  POutMin=[]  POutMax=[]  IOutMin=[]  IOutMax=[]  DOutMin=[]  DOutMax=[]  NOutMin=[]  NOutMax=[]  SumOutMin=[]  SumOutMax=[]  SaturationOutMin=[]  SaturationOutMax=[]  PParamMin=[]  PParamMax=[]  IParamMin=[]  IParamMax=[]  DParamMin=[]  DParamMax=[]  NParamMin=[]  NParamMax=[]  KbParamMin=[]  KbParamMax=[]  KtParamMin=[]  KtParamMax=[]  KbOutMin=[]  KbOutMax=[]  KtOutMin=[]  KtOutMax=[]  IntegratorOutMin=[]  IntegratorOutMax=[]  FilterOutMin=[]  FilterOutMax=[]  SumI1OutMin=[]  SumI1OutMax=[]  SumI2OutMin=[]  SumI2OutMax=[]  SumI3OutMin=[]  SumI3OutMax=[]  SumI4OutMin=[]  SumI4OutMax=[]  SumDOutMin=[]  SumDOutMax=[]  DifferentiatorOutMin=[]  DifferentiatorOutMax=[]  FilterDiffOutCoefMin=[]  FilterDiffOutCoefMax=[]  ReciprocalOutMin=[]  ReciprocalOutMax=[]  SumDenOutMin=[]  SumDenOutMax=[]  SumNumOutMin=[]  SumNumOutMax=[]  DivideOutMin=[]  DivideOutMax=[]  IntegratorContinuousStateAttributes=''  IntegratorStateMustResolveToSignalObject=off  IntegratorRTWStateStorageClass=Auto  FilterContinuousStateAttributes=''  FilterStateMustResolveToSignalObject=off  FilterRTWStateStorageClass=Auto  ParallelPVariant=InternalParameters  IdealPVariant=Disabled  IVariant=InternalParameters  DVariant=InternalParameters  IntegratorVariant=Continuous  SatVariant=Disabled  AWVariant=Passthrough  PCopyVariant=Disabled  TRVariant=Disabled  FdbkBlocksVariant=Forward  IdealPFdbkVariant=Disabled  SatFdbkVariant=Disabled  DerivativeFilterVariant=ContFilter  NVariant=InternalParameters  NCopyVariant=Disabled  FilterICVariant=InternalICsFilter  IntegratorICVariant=InternalICs  ExternalResetVariant=Disabled  TRSumVariant=Passthrough  SumFdbkVariant=Disabled  SumVariant=Sum_PID
  角速度闭环 : Scope  NumInputPorts=2
  设定值滤波 : Subsystem  mask{Frq=0.5, Order=2}
      mask prompts: Frq "Frq_Set"; Order "Order_Set"
  左推进方向 : Outport
  右推进方向 : Outport  Port=2
  左电机扭矩 : Outport  Port=3
  右电机扭矩 : Outport  Port=4
  wires:
  角速度PID/1 -> 推力解算/2(转向扭矩), 舵朝向指令/2(设定扭矩), 舵内缩指令/2(设定扭矩)
  角度反馈/1 -> Gain1/1
  Sum1/1 -> 推力分配/1(左右和)
  舵朝向指令/1(左右角度和) -> 方向分配/1(左右和)
  推力解算/1(左推力) -> Sum2/1, Sum1/1
  前进速度反馈/1 -> 前进速度控制/1(速度反馈), 前进速度闭环/1  "速度反馈"
  Sum2/1 -> 推力分配/2(左右差)
  前进速度控制/1(前进力输出) -> 前进速度闭环/2, 推力解算/1(前进力), 舵内缩指令/1(设定前进力), 舵朝向指令/1(设定前进力)  "前进力"
  船头方向PID/1(角速度) -> Sum/2, 角速度闭环/2  "角速度设定"
  推力分配/2(右推力) -> 右电机控制/2(推力设定), 推力设定/2  "右推力设定"
  推力解算/2(右推力) -> Sum2/2, Sum1/2
  推力分配/1(左推力) -> 左电机控制/2(推力设定), 推力设定/1  "左推力设定"
  左电机控制/1(设定扭矩) -> 左电机扭矩/1
  左电机转速反馈/1 -> 左电机控制/1(转速反馈)
  Rate Limiter/1 -> 设定值滤波/1(Signal)
  前进速度设定/1 -> 前进速度控制/2(速度设定)
  方向分配/2(右方向) -> 右推进方向/1
  设定值滤波/1(Output) -> 船头方向闭环/2, 船头方向PID/2(角度设定)  "角度设定"
  舵内缩指令/1(左右角度差) -> 方向分配/2(左右差)
  方向分配/1(左方向) -> 左推进方向/1
  角速度反馈/1 -> 角速度闭环/1, Sum/1  "角速度反馈"
  Sum/1 -> 角速度PID/1
  右电机控制/1(设定扭矩) -> 右电机扭矩/1
  侧移速度反馈/1 -> Scope3/1
  推进方向反馈/1 -> 推力解算/3(左右推进偏角)
  右电机转速反馈/1 -> 右电机控制/1(转速反馈)
  Gain1/1 -> 船头方向闭环/1, 船头方向PID/1(角度反馈)  "角度反馈"
  船头方向设定/1 -> Rate Limiter/1

== system propeller/失败的水流估计模型/水流状态估计/微分前滤波 ==
  Signal : Inport
  Constant2 : Constant  Value=Frq
  Gain : Gain  Gain=2*pi
  d_Smp_LPF6 : cstblocks/Linear Parameter Varying/Varying Lowpass Filter  N=Order
      settings: SourceProductName=Control System Toolbox
  Output : Outport
  wires:
  Gain/1 -> d_Smp_LPF6/2
  Signal/1 -> d_Smp_LPF6/1
  Constant2/1 -> Gain/1
  d_Smp_LPF6/1 -> Output/1  "Is"

== system propeller/失败的水流估计模型/水流状态估计/滞后1 ==
  Signal : Inport
  Constant2 : Constant  Value=Frq
  Gain : Gain  Gain=2*pi
  d_Smp_LPF6 : cstblocks/Linear Parameter Varying/Varying Lowpass Filter  N=Order
      settings: SourceProductName=Control System Toolbox
  Output : Outport
  wires:
  d_Smp_LPF6/1 -> Output/1  "Is"
  Constant2/1 -> Gain/1
  Signal/1 -> d_Smp_LPF6/1
  Gain/1 -> d_Smp_LPF6/2

== system propeller/失败的水流估计模型/水流状态估计/滞后2 ==
  Signal : Inport
  Constant2 : Constant  Value=Frq
  Gain : Gain  Gain=2*pi
  d_Smp_LPF6 : cstblocks/Linear Parameter Varying/Varying Lowpass Filter  N=Order
      settings: SourceProductName=Control System Toolbox
  Output : Outport
  wires:
  Gain/1 -> d_Smp_LPF6/2
  Signal/1 -> d_Smp_LPF6/1
  Constant2/1 -> Gain/1
  d_Smp_LPF6/1 -> Output/1  "Is"

== system propeller/失败的水流估计模型/水流状态估计/滞后3 ==
  Signal : Inport
  Constant2 : Constant  Value=Frq
  Gain : Gain  Gain=2*pi
  d_Smp_LPF6 : cstblocks/Linear Parameter Varying/Varying Lowpass Filter  N=Order
      settings: SourceProductName=Control System Toolbox
  Output : Outport
  wires:
  d_Smp_LPF6/1 -> Output/1  "Is"
  Constant2/1 -> Gain/1
  Signal/1 -> d_Smp_LPF6/1
  Gain/1 -> d_Smp_LPF6/2

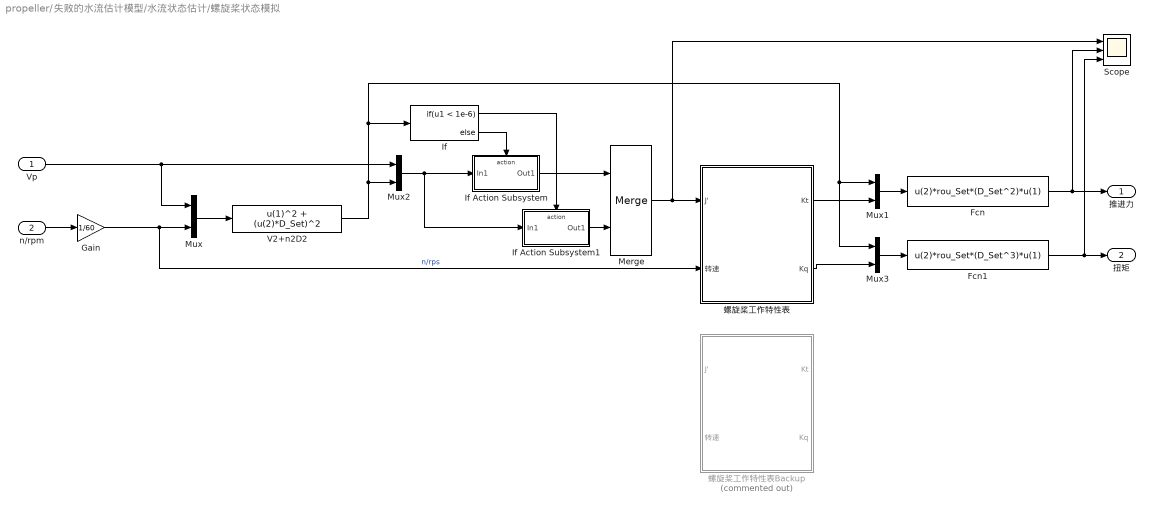
== system propeller/失败的水流估计模型/水流状态估计/螺旋桨状态模拟 ==
  Vp : Inport
  n/rpm : Inport  Port=2
  Fcn : Fcn  Expr=u(2)*rou_Set*(D_Set^2)*u(1)
  Fcn1 : Fcn  Expr=u(2)*rou_Set*(D_Set^3)*u(1)
  Gain : Gain  Gain=1/60
  If : If  IfExpression=u1 < 1e-6
  If Action Subsystem : Subsystem  TreatAsAtomicUnit=on
  If Action Subsystem1 : Subsystem  TreatAsAtomicUnit=on
  Merge : Merge
  Mux{,1..3} (4 alike) : Mux  Inputs=2
  Scope : Scope  NumInputPorts=3
  V2+n2D2 : Fcn  Expr=u(1)^2 + (u(2)*D_Set)^2
  螺旋桨工作特性表 : Subsystem
  螺旋桨工作特性表Backup : Subsystem  Commented=on
  推进力 : Outport
  扭矩 : Outport  Port=2
  wires:
  Fcn/1 -> 推进力/1, Scope/2
  Fcn1/1 -> 扭矩/1, Scope/3
  Mux3/1 -> Fcn1/1
  V2+n2D2/1 -> Mux2/2, Mux1/1, Mux3/1, If/1
  Mux1/1 -> Fcn/1
  螺旋桨工作特性表/2(Kq) -> Mux3/2
  螺旋桨工作特性表/1(Kt) -> Mux1/2
  Merge/1 -> 螺旋桨工作特性表/1(J'), Scope/1
  Mux/1 -> V2+n2D2/1
  If Action Subsystem1/1(Out1) -> Merge/2
  If/1 -> If Action Subsystem1/Action
  Gain/1 -> 螺旋桨工作特性表/2(转速), Mux/2  "n/rps"
  If Action Subsystem/1(Out1) -> Merge/1
  If/2 -> If Action Subsystem/Action
  Vp/1 -> Mux/1, Mux2/1
  n/rpm/1 -> Gain/1
  Mux2/1 -> If Action Subsystem/1(In1), If Action Subsystem1/1(In1)

== system propeller/失败的水流估计模型/水流状态估计/设定扭矩滤波1 ==
  Signal : Inport
  Constant2 : Constant  Value=Frq
  Gain : Gain  Gain=2*pi
  d_Smp_LPF6 : cstblocks/Linear Parameter Varying/Varying Lowpass Filter  N=Order
      settings: SourceProductName=Control System Toolbox
  Output : Outport
  wires:
  d_Smp_LPF6/1 -> Output/1  "Is"
  Constant2/1 -> Gain/1
  Signal/1 -> d_Smp_LPF6/1
  Gain/1 -> d_Smp_LPF6/2

== system propeller/失败的水流估计模型/水流状态估计/设定扭矩滤波2 ==
  Signal : Inport
  Constant2 : Constant  Value=Frq
  Gain : Gain  Gain=2*pi
  d_Smp_LPF6 : cstblocks/Linear Parameter Varying/Varying Lowpass Filter  N=Order
      settings: SourceProductName=Control System Toolbox
  Output : Outport
  wires:
  Gain/1 -> d_Smp_LPF6/2
  Signal/1 -> d_Smp_LPF6/1
  Constant2/1 -> Gain/1
  d_Smp_LPF6/1 -> Output/1  "Is"

== system propeller/失败的水流估计模型/螺旋桨模型/If Action Subsystem ==
  In1 : Inport
  Action Port : ActionPort  ActionPortLabel=else
  Fcn2 : Fcn  Expr=u(1)/(sqrt(u(2)))
  Out1 : Outport
  wires:
  In1/1 -> Fcn2/1
  Fcn2/1 -> Out1/1

== system propeller/失败的水流估计模型/螺旋桨模型/If Action Subsystem1 ==
  In1 : Inport
  Action Port : ActionPort  ActionPortLabel=if(u1 < 1e-6)
  Fcn2 : Fcn  Expr=abs(u(1))
  Out1 : Outport
  wires:
  Fcn2/1 -> Out1/1
  In1/1 -> Fcn2/1

== system propeller/失败的水流估计模型/螺旋桨模型/螺旋桨工作特性表 ==
  J' : Inport
  转速 : Inport  Port=2
  If Action Subsystem2 : Subsystem  TreatAsAtomicUnit=on
  If Action Subsystem3 : Subsystem  TreatAsAtomicUnit=on
  If1 : If
  Merge1 : Merge
  Merge2 : Merge
  Kt : Outport
  Kq : Outport  Port=2
  wires:
  If1/1 -> If Action Subsystem2/Action
  If1/2 -> If Action Subsystem3/Action
  转速/1 -> If1/1
  If Action Subsystem2/1(Kt) -> Merge1/1
  J'/1 -> If Action Subsystem3/1(J'), If Action Subsystem2/1(J')
  Merge1/1 -> Kt/1
  If Action Subsystem3/1(Kt) -> Merge1/2
  If Action Subsystem3/2(Kq) -> Merge2/2
  Merge2/1 -> Kq/1
  If Action Subsystem2/2(Kq) -> Merge2/1

== system propeller/失败的水流估计模型/螺旋桨模型/螺旋桨工作特性表Backup ==
  J' : Inport
  转速 : Inport  Port=2
  If Action Subsystem2 : Subsystem  TreatAsAtomicUnit=on
  If Action Subsystem3 : Subsystem  TreatAsAtomicUnit=on
  If1 : If
  Merge1 : Merge
  Merge2 : Merge
  Kt : Outport
  Kq : Outport  Port=2
  wires:
  If Action Subsystem2/2(Kq) -> Merge2/1
  Merge2/1 -> Kq/1
  If Action Subsystem3/2(Kq) -> Merge2/2
  If Action Subsystem3/1(Kt) -> Merge1/2
  Merge1/1 -> Kt/1
  J'/1 -> If Action Subsystem2/1(J'), If Action Subsystem3/1(J')
  If Action Subsystem2/1(Kt) -> Merge1/1
  转速/1 -> If1/1
  If1/2 -> If Action Subsystem3/Action
  If1/1 -> If Action Subsystem2/Action

== system propeller/失败的水流估计模型/预期转速计算/滞后2 ==
  Signal : Inport
  Constant2 : Constant  Value=Frq
  Gain : Gain  Gain=2*pi
  d_Smp_LPF6 : cstblocks/Linear Parameter Varying/Varying Lowpass Filter  N=Order
      settings: SourceProductName=Control System Toolbox
  Output : Outport
  wires:
  Gain/1 -> d_Smp_LPF6/2
  Signal/1 -> d_Smp_LPF6/1
  Constant2/1 -> Gain/1
  d_Smp_LPF6/1 -> Output/1  "Is"

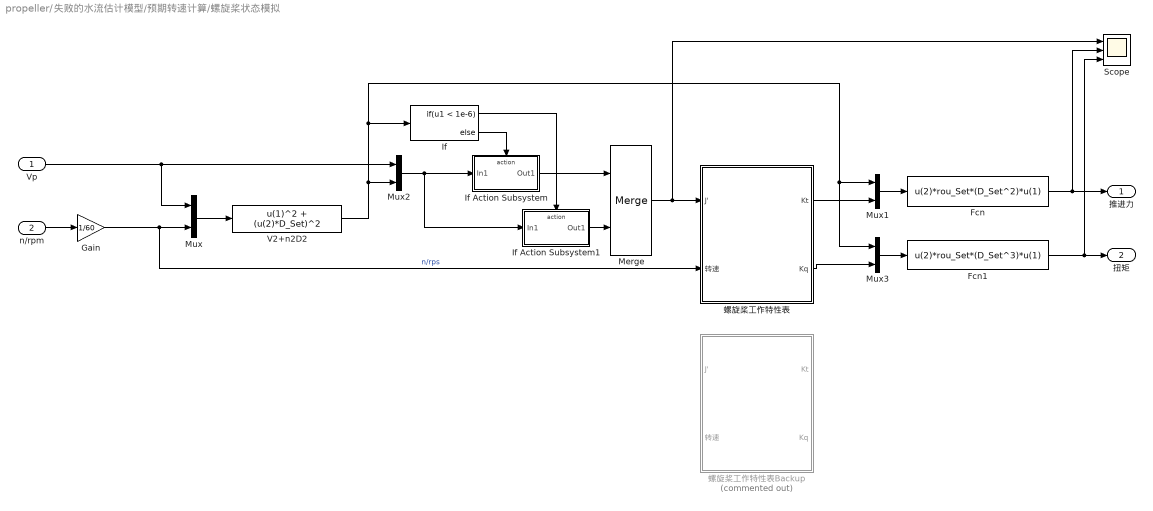
== system propeller/失败的水流估计模型/预期转速计算/螺旋桨状态模拟 ==
  Vp : Inport
  n/rpm : Inport  Port=2
  Fcn : Fcn  Expr=u(2)*rou_Set*(D_Set^2)*u(1)
  Fcn1 : Fcn  Expr=u(2)*rou_Set*(D_Set^3)*u(1)
  Gain : Gain  Gain=1/60
  If : If  IfExpression=u1 < 1e-6
  If Action Subsystem : Subsystem  TreatAsAtomicUnit=on
  If Action Subsystem1 : Subsystem  TreatAsAtomicUnit=on
  Merge : Merge
  Mux{,1..3} (4 alike) : Mux  Inputs=2
  Scope : Scope  NumInputPorts=3
  V2+n2D2 : Fcn  Expr=u(1)^2 + (u(2)*D_Set)^2
  螺旋桨工作特性表 : Subsystem
  螺旋桨工作特性表Backup : Subsystem  Commented=on
  推进力 : Outport
  扭矩 : Outport  Port=2
  wires:
  Fcn/1 -> 推进力/1, Scope/2
  Fcn1/1 -> 扭矩/1, Scope/3
  Mux3/1 -> Fcn1/1
  V2+n2D2/1 -> Mux2/2, Mux1/1, Mux3/1, If/1
  Mux1/1 -> Fcn/1
  螺旋桨工作特性表/2(Kq) -> Mux3/2
  螺旋桨工作特性表/1(Kt) -> Mux1/2
  Merge/1 -> 螺旋桨工作特性表/1(J'), Scope/1
  Mux/1 -> V2+n2D2/1
  If Action Subsystem1/1(Out1) -> Merge/2
  If/1 -> If Action Subsystem1/Action
  Gain/1 -> 螺旋桨工作特性表/2(转速), Mux/2  "n/rps"
  If Action Subsystem/1(Out1) -> Merge/1
  If/2 -> If Action Subsystem/Action
  Vp/1 -> Mux/1, Mux2/1
  n/rpm/1 -> Gain/1
  Mux2/1 -> If Action Subsystem/1(In1), If Action Subsystem1/1(In1)

== system propeller/失败的水流估计模型/驱动电机/反馈量滤波 ==
  Signal : Inport
  Constant2 : Constant  Value=Frq
  Gain : Gain  Gain=2*pi
  d_Smp_LPF6 : cstblocks/Linear Parameter Varying/Varying Lowpass Filter  N=Order
      settings: SourceProductName=Control System Toolbox
  Output : Outport
  wires:
  Gain/1 -> d_Smp_LPF6/2
  Signal/1 -> d_Smp_LPF6/1
  Constant2/1 -> Gain/1
  d_Smp_LPF6/1 -> Output/1  "Is"

== system propeller/失败的水流估计模型/驱动电机/滞后 ==
  Signal : Inport
  Constant2 : Constant  Value=Frq
  Gain : Gain  Gain=2*pi
  d_Smp_LPF6 : cstblocks/Linear Parameter Varying/Varying Lowpass Filter  N=Order
      settings: SourceProductName=Control System Toolbox
  Output : Outport
  wires:
  Gain/1 -> d_Smp_LPF6/2
  Signal/1 -> d_Smp_LPF6/1
  Constant2/1 -> Gain/1
  d_Smp_LPF6/1 -> Output/1  "Is"

== system propeller/直接转矩控制/GPS船速/反馈量滤波 ==
  Signal : Inport
  Constant2 : Constant  Value=Frq
  Gain : Gain  Gain=2*pi
  d_Smp_LPF6 : cstblocks/Linear Parameter Varying/Varying Lowpass Filter  N=Order
      settings: SourceProductName=Control System Toolbox
  Output : Outport
  wires:
  Gain/1 -> d_Smp_LPF6/2
  Signal/1 -> d_Smp_LPF6/1
  Constant2/1 -> Gain/1
  d_Smp_LPF6/1 -> Output/1  "Is"

== system propeller/直接转矩控制/GPS船速/反馈量滤波1 ==
  Signal : Inport
  Constant2 : Constant  Value=Frq
  Gain : Gain  Gain=2*pi
  d_Smp_LPF6 : cstblocks/Linear Parameter Varying/Varying Lowpass Filter  N=Order
      settings: SourceProductName=Control System Toolbox
  Output : Outport
  wires:
  Gain/1 -> d_Smp_LPF6/2
  Signal/1 -> d_Smp_LPF6/1
  Constant2/1 -> Gain/1
  d_Smp_LPF6/1 -> Output/1  "Is"

== system propeller/直接转矩控制/船体、水体物理模型/Multibody ==
  Mechanism Configuration : sm_lib/Utilities/Mechanism Configuration  UniformGravity=Constant  GravityVector=[0 0 -9.80665]  GravityUnits=m/s^2  LinearizationDelta=0.001
  Solver Configuration : nesl_utility/Solver Configuration  PhysicalDomain=network_engine_domain  SubClassName=solver  LeftPortType=input  RightPortType=generic  Tones=[]  Harmonics=[]  SimulateNoise=off  Profile=off  UseLocalSampling=off  EnableSwitchedLinearOptims=on  FrequencyDomain=off  UseCCode=off  RelTol=0.001  AbsTol=1e-06  MinStep=1e-09  ToWorkspace=off  RevertToSquareIcSolve=off  NumHomotopyIterations=100  PhasorMode=off  PhasorModeNumHarmonics=1  DoDC=off  ResidualTolerance=1e-09  UseLocalSolver=off  LocalSolverChoice=NE_BACKWARD_EULER_ADVANCER  LocalSolverSampleTime=0.001  DoFixedCost=off  MaxNonlinIter=3  MaxModeIter=2  LinearAlgebra=Sparse  EquationFormulation=NE_TIME_EF  DelaysMemoryBudget=1024  AutomaticFiltering=on  FilteringTimeConstant=0.001  PartitionStorageMethod=AS_NEEDED  PartitionMemoryBudget=1024  PartitionMethod=FAST
  World Frame : sm_lib/Frames and Transforms/World Frame
  大地系 : PMIOPort  Side=Right
  connections:
  Solver Configuration/RConn1 -- 大地系/RConn1 -- World Frame/RConn1 -- Mechanism Configuration/RConn1

== system propeller/直接转矩控制/船体、水体物理模型/对水船速 ==
  Vx : Inport
  Vy : Inport  Port=2
  Alpha : Inport  Port=3
  Fcn1 : Fcn  Expr=u(2)*cos(u(3))-u(1)*sin(u(3))
  Fcn2 : Fcn  Expr=u(2)*sin(u(3))+u(1)*cos(u(3))
  Mux1 : Mux  Inputs=3
  纵向速度 : Outport
  横向速度 : Outport  Port=2
  wires:
  Fcn2/1 -> 横向速度/1
  Mux1/1 -> Fcn2/1, Fcn1/1
  Vy/1 -> Mux1/2
  Vx/1 -> Mux1/1
  Alpha/1 -> Mux1/3
  Fcn1/1 -> 纵向速度/1

== system propeller/直接转矩控制/船体、水体物理模型/推进器1 ==
  推进器偏角 : Inport
  横向船速 : Inport  Port=2
  纵向船速 : Inport  Port=3
  设定扭矩 : Inport  Port=4
  Fcn1 : Fcn  Expr=u(1)*(1-u(2))
  Fcn2 : Fcn  Expr=u(2)*cos(u(3))-u(1)*sin(u(3))
  Memory1 : Memory
  Mux1 : Mux  Inputs=2
  Mux2 : Mux  Inputs=3
  Scope : Scope  NumInputPorts=2
  Zero-Order Hold1 : ZeroOrderHold  SampleTime=0.05
  伴流分数 : Constant  Value=0.1
  螺旋桨模型 : Subsystem  mask{rou_Set=1.023, D_Set=1}
      mask prompts: rou_Set "海水密度 g/cm3 (rou_Set)"; D_Set "螺旋桨直径 D_Set"
  驱动电机 : Subsystem  mask{Trq_Max=250, Spe_Max=20000, J_Set=0.1}
      mask prompts: Trq_Max "电机最大扭矩"; Spe_Max "电机最高转速"; J_Set "系统转动惯量"
  实际推力 : Outport
  转速反馈 : Outport  Port=2
  wires:
  Mux2/1 -> Fcn2/1
  Mux1/1 -> Fcn1/1
  驱动电机/2(转速反馈) -> 转速反馈/1  "转速反馈"
  Fcn1/1 -> Zero-Order Hold1/1
  Fcn2/1 -> Mux1/1  "对水速度"
  螺旋桨模型/2(扭矩) -> 驱动电机/1(实际负载扭矩)
  驱动电机/1(实际转速) -> 螺旋桨模型/2(n/rpm)
  伴流分数/1 -> Mux1/2
  推进器偏角/1 -> Mux2/3
  纵向船速/1 -> Mux2/2
  横向船速/1 -> Mux2/1
  螺旋桨模型/1(推进力) -> 实际推力/1, Scope/2
  Zero-Order Hold1/1 -> Memory1/1
  Memory1/1 -> 螺旋桨模型/1(Vp), Scope/1
  设定扭矩/1 -> 驱动电机/2(设定扭矩)

== system propeller/直接转矩控制/船体、水体物理模型/推进器2 ==
  推进器偏角 : Inport
  横向船速 : Inport  Port=2
  纵向船速 : Inport  Port=3
  设定扭矩 : Inport  Port=4
  Fcn1 : Fcn  Expr=u(1)*(1-u(2))
  Fcn2 : Fcn  Expr=u(2)*cos(u(3))-u(1)*sin(u(3))
  Memory1 : Memory
  Mux1 : Mux  Inputs=2
  Mux2 : Mux  Inputs=3
  Scope : Scope  NumInputPorts=2
  Zero-Order Hold1 : ZeroOrderHold  SampleTime=0.05
  伴流分数 : Constant  Value=0.1
  螺旋桨模型 : Subsystem  mask{rou_Set=1.023, D_Set=1}
      mask prompts: rou_Set "海水密度 g/cm3 (rou_Set)"; D_Set "螺旋桨直径 D_Set"
  驱动电机 : Subsystem  mask{Trq_Max=250, Spe_Max=20000, J_Set=0.1}
      mask prompts: Trq_Max "电机最大扭矩"; Spe_Max "电机最高转速"; J_Set "系统转动惯量"
  实际推力 : Outport
  转速反馈 : Outport  Port=2
  wires:
  设定扭矩/1 -> 驱动电机/2(设定扭矩)
  Memory1/1 -> Scope/1, 螺旋桨模型/1(Vp)
  Zero-Order Hold1/1 -> Memory1/1
  螺旋桨模型/1(推进力) -> Scope/2, 实际推力/1
  横向船速/1 -> Mux2/1
  纵向船速/1 -> Mux2/2
  推进器偏角/1 -> Mux2/3
  伴流分数/1 -> Mux1/2
  驱动电机/1(实际转速) -> 螺旋桨模型/2(n/rpm)
  螺旋桨模型/2(扭矩) -> 驱动电机/1(实际负载扭矩)
  Fcn2/1 -> Mux1/1  "对水速度"
  Fcn1/1 -> Zero-Order Hold1/1
  驱动电机/2(转速反馈) -> 转速反馈/1  "转速反馈"
  Mux1/1 -> Fcn1/1
  Mux2/1 -> Fcn2/1

== system propeller/直接转矩控制/船体、水体物理模型/水流设置 ==
  Vx_In : Inport
  Vy_In : Inport  Port=2
  Complex to Real-Imag : ComplexToRealImag
  Gain : Gain  Gain=pi/180
  Magnitude-Angle to Complex : MagnitudeAngleToComplex
  Real-Imag to Complex : RealImagToComplex
  Sum : Sum  Inputs=|+-
  流速 : Constant  Value=Spe
  角度 : Constant  Value=Dir
  Vx_Out : Outport
  Vy_Out : Outport  Port=2
  wires:
  Sum/1 -> Complex to Real-Imag/1  "对水速度"
  流速/1 -> Magnitude-Angle to Complex/1
  Magnitude-Angle to Complex/1 -> Sum/2  "水流速度"
  Gain/1 -> Magnitude-Angle to Complex/2
  角度/1 -> Gain/1
  Vy_In/1 -> Real-Imag to Complex/2
  Real-Imag to Complex/1 -> Sum/1  "对地速度"
  Complex to Real-Imag/2 -> Vy_Out/1
  Complex to Real-Imag/1 -> Vx_Out/1
  Vx_In/1 -> Real-Imag to Complex/1

== system propeller/直接转矩控制/船体、水体物理模型/水阻计算 ==
  纵向船速 : Inport
  横向船速 : Inport  Port=2
  船体角速度 : Inport  Port=3
  Product : Product
  Product1 : Product
  Product2 : Product
  Sign : Signum
  Sign1 : Signum
  Sign2 : Signum
  旋转水阻表达式 : Fcn  Expr=-u^2*K_z
  横向水阻表达式 : Fcn  Expr=-u^2*K_x
  纵向水阻表达式 : Fcn  Expr=-u^2*K_y
  纵向水阻 : Outport
  横向水阻 : Outport  Port=2
  旋转水阻 : Outport  Port=3
  wires:
  纵向船速/1 -> Sign/1, 纵向水阻表达式/1
  横向船速/1 -> Sign1/1, 横向水阻表达式/1
  船体角速度/1 -> Sign2/1, 旋转水阻表达式/1
  纵向水阻表达式/1 -> Product/2  "纵向水阻"
  Sign/1 -> Product/1
  横向水阻表达式/1 -> Product1/2  "横向水阻"
  Sign1/1 -> Product1/1
  Sign2/1 -> Product2/1
  旋转水阻表达式/1 -> Product2/2  "旋转水阻"
  Product2/1 -> 旋转水阻/1
  Product1/1 -> 横向水阻/1
  Product/1 -> 纵向水阻/1
